simulink model "FP_250521"  (R2024a)
settings: Solver=VariableStepAuto  StartTime=0.0  StopTime=10.0  RelTol=1e-3
values from neighbouring files (symbols this model uses):
  global_path_xy_dense = [-80.8928520527 -80.3602143869 -79.8516651737 -79.3645247642 -78.8961135098 -78.4437517617 -78.004759871 -77.5764581893 -77.1561670675 -76.7412068571 -76.3288979094 -75.9165605754 ... (728 elements, 364x2)]    [global_path_xy_dense_y-34.mat]
undefined symbols (not defined in the file or in its folder): Do_waypoints, do_waypoints_tail_shifted, pathXY, route1_waypoint, route1_waypoint_raw, route2_waypoint, route2_waypoint_raw, route3_waypoint, route3_waypoint_raw
libraries: CarMaker4SL x192, slpidlib x4
(part 4 of 4)

== matlab function FP_250521/Final Project3/Scenario 1/MATLAB Function4  ==
  settings: updateMethod=DISCRETE  sampleTime=0.05
  data: waypoints input; local_waypoints_ output; vehicle_position input; head input
% function local_waypoints_ = global_to_local_waypoints(waypoints, vehicle_position, head)
%     N = size(waypoints, 1);
%     local_waypoints_ = zeros(N, 2);
% 
%     % 이동 평균 필터 윈도우 크기 설정
%     window_size = 65;
% 
% 
%     % 이동 평균 필터 적용 (x, y 각각)
%     x_filtered = movmean(waypoints(:,1), window_size);
%     y_filtered = movmean(waypoints(:,2), window_size);
% 
%     % 좌표계 변환을 위한 cos/sin
%     cos_yaw = cos(-head);
%     sin_yaw = sin(-head);
% 
%     for i = 1:N
%         dx = x_filtered(i) - vehicle_position(1);
%         dy = y_filtered(i) - vehicle_position(2);
% 
%         local_x = dx * cos_yaw - dy * sin_yaw;
%         local_y = dx * sin_yaw + dy * cos_yaw;
% 
%         local_waypoints_(i,1) = local_x;
%         local_waypoints_(i,2) = local_y;
%     end
% end

function local_waypoints_ = global_to_local_waypoints(waypoints, vehicle_position, head)
    N = size(waypoints, 1);
    local_waypoints_ = zeros(N, 2);

    window_size_main = 65;    % 기본 윈도우
    window_size_tail = 20;    % 꼬리(마지막 70개 구간) 윈도우

    x_filtered = zeros(N,1);
    y_filtered = zeros(N,1);

    for i = 1:N
        % 마지막 70개 전부터 윈도우 크기 30 적용
        if i > N - 70
            w = window_size_tail;
        else
            w = window_size_main;
        end
        % 윈도우 중앙 기준: [i - left, i + right] 범위
        half_win = floor(w/2);
        idx1 = max(1, i - half_win);
        idx2 = min(N, i + half_win);
        x_filtered(i) = mean(waypoints(idx1:idx2, 1));
        y_filtered(i) = mean(waypoints(idx1:idx2, 2));
    end

    % 좌표계 변환
    cos_yaw = cos(-head);
    sin_yaw = sin(-head);

    for i = 1:N
        dx = x_filtered(i) - vehicle_position(1);
        dy = y_filtered(i) - vehicle_position(2);

        local_x = dx * cos_yaw - dy * sin_yaw;
        local_y = dx * sin_yaw + dy * cos_yaw;

        local_waypoints_(i,1) = local_x;
        local_waypoints_(i,2) = local_y;
    end
end

== matlab function FP_250521/Final Project3/Scenario 1/MATLAB Function9 ==
  settings: updateMethod=DISCRETE  sampleTime=0.05
  data: ego_pos input; traffic_info input; ego_lane_idx output; wp1 input; wp2 input; wp3 input; traffic_lane_idx output
function [ego_lane_idx, traffic_lane_idx] = get_lane_indices_split(ego_pos, traffic_info, wp1, wp2, wp3)
% ego_pos: [1 x 2]
% traffic_info: [8 x 10] → 각 행: [x, y, vx, vy, ax, ay, yaw, yawRate, length, width]
% wp1~3: [N x 2] (차선별 waypoint 좌표)
% ego_lane_idx: 자차 차선 번호 (1~3)
% traffic_lane_idx: [8 x 1] (각 차량의 차선 번호)

    traffic_pos = traffic_info(:, 1:2);  % x, y 추출
    num_traffic = size(traffic_pos, 1);  % 8 expected
    traffic_lane_idx = zeros(num_traffic, 1);

    % 거리 계산 함수
    function d = min_dist(p, wp)
        dx = wp(:,1) - p(1);
        dy = wp(:,2) - p(2);
        d = min(sqrt(dx.^2 + dy.^2));
    end

    % 자차 차선 판단
    d1 = min_dist(ego_pos, wp1);
    d2 = min_dist(ego_pos, wp2);
    d3 = min_dist(ego_pos, wp3);
    [~, ego_lane_idx] = min([d1, d2, d3]);

    % 트래픽 차량들 차선 판단
    for i = 1:num_traffic
        car_pos = traffic_pos(i, :);
        d1 = min_dist(car_pos, wp1);
        d2 = min_dist(car_pos, wp2);
        d3 = min_dist(car_pos, wp3);
        [~, traffic_lane_idx(i)] = min([d1, d2, d3]);
    end
end

== matlab function FP_250521/Final Project3/Scenario 1/MATLAB Function ==
  data: u1 input; y output; u2 input
function y = and_logic_latch_permanent(u1, u2)
%#codegen
persistent latch;
if isempty(latch)
    latch = 0;
end

% 정지 조건에 한 번이라도 들어가면 latch=1이 되고, 이후엔 절대 복귀하지 않음
if (u1 > 5) && (u1 < 6) && (u2 > -38) && (u2 < -35)
    latch = 1;
end

y = latch;
end

== matlab function FP_250521/Final Project1/Scenario 1/MATLAB Function11 ==
  settings: updateMethod=DISCRETE  sampleTime=0.05
  data: ego_pos input; ego_yaw input; ego_vx input; ego_lane_idx input; traffic_info input; target_speed output; traffic_lane_idx input; debug_dist output
% function [target_speed, debug_dist] = acc_target_speed_global_based( ...
%     ego_pos, ego_yaw, ego_vx, ego_lane_idx, ...
%     traffic_info, traffic_lane_idx)
% 
%     % 기본 설정
%     default_speed = 16.0;   % m/s
%     min_gap = 20;           % 최소 안전 거리
%     max_gap = 35;           % 거리 완충 구간
% 
%     % === traffic_info: [8x10] ===
%     % 컬럼:
%     % 1: x, 2: y, 3: vx, 4: vy, 5: ax, 6: ay, 7: yaw, 8: yawrate, 9: len, 10: width
%     traffic_pos = traffic_info(:, 1:2);  % [8x2]
%     traffic_vx = traffic_info(:, 3);     % [8x1]
% 
%     L = size(traffic_info, 1);  % 차량 수 (8)
% 
%     min_dist = inf;
%     front_vx = 0;
%     found = false;
% 
%     % Ego 진행 방향 단위벡터
%     ego_dir = [cos(ego_yaw); sin(ego_yaw)];
% 
%     for i = 1:L
%         if traffic_lane_idx(i) == ego_lane_idx
%             dx = traffic_pos(i,1) - ego_pos(1);
%             dy = traffic_pos(i,2) - ego_pos(2);
%             rel_vec = [dx; dy];
% 
%             % 전방 차량인지 판단
%             if dot(rel_vec, ego_dir) > 0
%                 dist = norm(rel_vec);
% 
%                 if dist < min_dist
%                     min_dist = dist;
%                     front_vx = traffic_vx(i);
%                     found = true;
%                 end
%             end
%         end
%     end
% 
%     % 속도 설정
%     target_speed = default_speed;
% 
%     if found
%         if min_dist < min_gap
%             target_speed = front_vx;
%         elseif min_dist < max_gap
%             ratio = (min_dist - min_gap) / (max_gap - min_gap);
%             target_speed = front_vx * ratio + default_speed * (1 - ratio);
%         else
%             target_speed = default_speed;
%         end
%     end
% 
%     debug_dist = min_dist;
% end



function [target_speed, debug_dist] = acc_target_speed_global_based( ...
    ego_pos, ego_yaw, ego_vx, ego_lane_idx, ...
    traffic_info, traffic_lane_idx)

    % 기본 설정
    default_speed = 18;   % m/s
    min_gap = 25;           % 최소 안전 거리
    max_gap = 50;           % 거리 완충 구간
    min_speed = 3.5;        % 최저속도(정지 방지)

    % === traffic_info: [8x10] ===
    % 1: x, 2: y, 3: vx, ...
    traffic_pos = traffic_info(:, 1:2);  % [8x2]
    traffic_vx = traffic_info(:, 3);     % [8x1]

    L = size(traffic_info, 1);  % 차량 수 (8)

    min_dist = inf;
    front_vx = 0;
    found = false;

    % Ego 진행 방향 단위벡터
    ego_dir = [cos(ego_yaw); sin(ego_yaw)];

    for i = 1:L
        if traffic_lane_idx(i) == ego_lane_idx
            dx = traffic_pos(i,1) - ego_pos(1);
            dy = traffic_pos(i,2) - ego_pos(2);
            rel_vec = [dx; dy];

            % 전방 차량인지 판단
            if dot(rel_vec, ego_dir) > 0
                dist = norm(rel_vec);

                if dist < min_dist
                    min_dist = dist;
                    front_vx = traffic_vx(i);
                    found = true;
                end
            end
        end
    end

    % 속도 설정
    target_speed = default_speed;

    if found
        % *** 디버깅 로그 출력 (필요시 주석 해제) ***
        % disp(['front_vx=', num2str(front_vx), ', min_dist=', num2str(min_dist)]);

        % front_vx가 비정상(음수/NaN/이상치)이거나 너무 작으면 방어!
        if isnan(front_vx) || front_vx < 0
            front_vx = min_speed;
        end

        if min_dist < min_gap
            % 앞차 속도가 0일 때만 내 차도 정지, 그 외엔 최소 속도 유지
            if front_vx <= min_speed
                target_speed = min_speed;
            else
                target_speed = front_vx;
            end
        elseif min_dist < max_gap
            ratio = (min_dist - min_gap) / (max_gap - min_gap);
            % 보간 결과가 너무 작을 경우도 방어
            blend_speed = front_vx * ratio + default_speed * (1 - ratio);
            target_speed = max(blend_speed, min_speed);
        else
            target_speed = default_speed;
        end
    end

    % 추가 방어: target_speed는 항상 min_speed 이상 보장
    target_speed = max(target_speed, min_speed);

    debug_dist = min_dist;
end

== matlab function FP_250521/Final Project1/Scenario 1/MATLAB Function3 ==
  settings: updateMethod=DISCRETE  sampleTime=0.05
  data: poly_coeff input; lateral_error output; velocity input; lookahead_time input; x_lookahead output; delta_ff output; dy output; d2y output; kappa output
function [lateral_error, x_lookahead, delta_ff, dy, d2y, kappa] = compute_lateral_error_(poly_coeff, velocity, lookahead_time)
% ------------------------------------------------------------
% 경로 다항식 기반 곡률 및 조향각 계산 (스무딩 포함)
% Waypoint 부족 시 조향각 0 처리
% ------------------------------------------------------------

% 휠베이스
L = 3.0;

% Waypoint 부족으로 poly_coeff가 모두 0일 경우 → 계산 중단
if all(poly_coeff == 0)
    lateral_error = 0;
    x_lookahead = velocity * lookahead_time;
    delta_ff = 0;
    dy = 0;
    d2y = 0;
    kappa = 0;
    return;
end

% 다항식 계수 추출
a = 0; b = 0; c = 0; d = 0;
n = length(poly_coeff);
if n == 4
    a = poly_coeff(1); b = poly_coeff(2); c = poly_coeff(3); d = poly_coeff(4);
elseif n == 3
    b = poly_coeff(1); c = poly_coeff(2); d = poly_coeff(3);
elseif n == 2
    c = poly_coeff(1); d = poly_coeff(2);
else
    d = poly_coeff(1);
end

% 1. lateral error (x = 0)
lateral_error = d;

% 2. lookahead 위치
x_lookahead = velocity * lookahead_time;

% 3. dy, d2y
dy = 3*a*x_lookahead^2 + 2*b*x_lookahead + c;
d2y = 6*a*x_lookahead + 2*b;

% 4. kappa 계산 (수치 안정성 보장)
denominator = (1 + dy^2)^(3/2);
if denominator < 1e-6
    denominator = 1e-6;
end
kappa = d2y / denominator;

% 5. 조향각 계산
delta_now = L * kappa;

% 6. Moving Average Filter 적용 (스무딩)
persistent delta_buffer
if isempty(delta_buffer)
    delta_buffer = zeros(1, 30);  % 최근 30개 저장
end

% shift + 최신값 추가
delta_buffer = [delta_now, delta_buffer(1:end-1)];

% 평균값 출력
delta_ff = mean(delta_buffer);

end

== matlab function FP_250521/Final Project1/Scenario 1/MATLAB Function4 ==
  settings: updateMethod=DISCRETE  sampleTime=0.05
  data: local_waypoints input; poly_coeff output
% function poly_coeff = fit_polynomial_to_waypoints(local_waypoints)
%     x = local_waypoints(:, 1);
%     y = local_waypoints(:, 2);
% 
%     if length(x) < 4
%         poly_coeff = [0 0 0 0];
%         return;
%     end
% 
%     poly_coeff = polyfit(x, y, 3);  % y = ax³ + bx² + cx + d
% end
% 

function poly_coeff = fit_polynomial_to_waypoints_(local_waypoints)

% 설정값
poly_order = 3;
max_points = 10;
x_limit = 20;
y_limit = 5;

% 1. x > 0, x < x_limit, |y| < y_limit 필터링
idx = find( ...
    local_waypoints(:,1) > 0 & ...
    local_waypoints(:,1) < x_limit & ...
    abs(local_waypoints(:,2)) < y_limit );

filtered = local_waypoints(idx, :);

% 2. 앞쪽 max_points개만 사용
N = min(max_points, size(filtered, 1));
x = filtered(1:N, 1);
y = filtered(1:N, 2);

% 3. 피팅 수행
if length(x) >= poly_order + 1
    poly_coeff = polyfit(x, y, poly_order);
else
    poly_coeff = zeros(1, 4);
end

end

== matlab function FP_250521/Final Project1/Scenario 1/MATLAB Function4  ==
  settings: updateMethod=DISCRETE  sampleTime=0.05
  data: waypoints input; local_waypoints_ output; vehicle_position input; head input
function local_waypoints_ = global_to_local_waypoints(waypoints, vehicle_position, head)
    N = size(waypoints, 1);
    local_waypoints_ = zeros(N, 2);

    % 이동 평균 필터 윈도우 크기 설정
    window_size = 65;


    % 이동 평균 필터 적용 (x, y 각각)
    x_filtered = movmean(waypoints(:,1), window_size);
    y_filtered = movmean(waypoints(:,2), window_size);

    % 좌표계 변환을 위한 cos/sin
    cos_yaw = cos(-head);
    sin_yaw = sin(-head);

    for i = 1:N
        dx = x_filtered(i) - vehicle_position(1);
        dy = y_filtered(i) - vehicle_position(2);

        local_x = dx * cos_yaw - dy * sin_yaw;
        local_y = dx * sin_yaw + dy * cos_yaw;

        local_waypoints_(i,1) = local_x;
        local_waypoints_(i,2) = local_y;
    end
end

== matlab function FP_250521/Final Project1/Scenario 1/MATLAB Function9 ==
  settings: updateMethod=DISCRETE  sampleTime=0.05
  data: ego_pos input; traffic_info input; ego_lane_idx output; wp1 input; wp2 input; wp3 input; traffic_lane_idx output
function [ego_lane_idx, traffic_lane_idx] = get_lane_indices_split(ego_pos, traffic_info, wp1, wp2, wp3)
% ego_pos: [1 x 2]
% traffic_info: [8 x 10] → 각 행: [x, y, vx, vy, ax, ay, yaw, yawRate, length, width]
% wp1~3: [N x 2] (차선별 waypoint 좌표)
% ego_lane_idx: 자차 차선 번호 (1~3)
% traffic_lane_idx: [8 x 1] (각 차량의 차선 번호)

    traffic_pos = traffic_info(:, 1:2);  % x, y 추출
    num_traffic = size(traffic_pos, 1);  % 8 expected
    traffic_lane_idx = zeros(num_traffic, 1);

    % 거리 계산 함수
    function d = min_dist(p, wp)
        dx = wp(:,1) - p(1);
        dy = wp(:,2) - p(2);
        d = min(sqrt(dx.^2 + dy.^2));
    end

    % 자차 차선 판단
    d1 = min_dist(ego_pos, wp1);
    d2 = min_dist(ego_pos, wp2);
    d3 = min_dist(ego_pos, wp3);
    [~, ego_lane_idx] = min([d1, d2, d3]);

    % 트래픽 차량들 차선 판단
    for i = 1:num_traffic
        car_pos = traffic_pos(i, :);
        d1 = min_dist(car_pos, wp1);
        d2 = min_dist(car_pos, wp2);
        d3 = min_dist(car_pos, wp3);
        [~, traffic_lane_idx(i)] = min([d1, d2, d3]);
    end
end

== matlab function FP_250521/Final Project3/Scenario 1/MATLAB Function11 ==
  settings: updateMethod=DISCRETE  sampleTime=0.05
  data: ego_pos input; ego_yaw input; ego_vx input; ego_lane_idx input; traffic_info input; target_speed output; traffic_lane_idx input; debug_dist output; global_x input; stop_flag output
% function [target_speed, debug_dist] = acc_target_speed_global_based( ...
%     ego_pos, ego_yaw, ego_vx, ego_lane_idx, ...
%     traffic_info, traffic_lane_idx)
% 
%     % 기본 설정
%     default_speed = 16.0;   % m/s
%     min_gap = 20;           % 최소 안전 거리
%     max_gap = 35;           % 거리 완충 구간
% 
%     % === traffic_info: [8x10] ===
%     % 컬럼:
%     % 1: x, 2: y, 3: vx, 4: vy, 5: ax, 6: ay, 7: yaw, 8: yawrate, 9: len, 10: width
%     traffic_pos = traffic_info(:, 1:2);  % [8x2]
%     traffic_vx = traffic_info(:, 3);     % [8x1]
% 
%     L = size(traffic_info, 1);  % 차량 수 (8)
% 
%     min_dist = inf;
%     front_vx = 0;
%     found = false;
% 
%     % Ego 진행 방향 단위벡터
%     ego_dir = [cos(ego_yaw); sin(ego_yaw)];
% 
%     for i = 1:L
%         if traffic_lane_idx(i) == ego_lane_idx
%             dx = traffic_pos(i,1) - ego_pos(1);
%             dy = traffic_pos(i,2) - ego_pos(2);
%             rel_vec = [dx; dy];
% 
%             % 전방 차량인지 판단
%             if dot(rel_vec, ego_dir) > 0
%                 dist = norm(rel_vec);
% 
%                 if dist < min_dist
%                     min_dist = dist;
%                     front_vx = traffic_vx(i);
%                     found = true;
%                 end
%             end
%         end
%     end
% 
%     % 속도 설정
%     target_speed = default_speed;
% 
%     if found
%         if min_dist < min_gap
%             target_speed = front_vx;
%         elseif min_dist < max_gap
%             ratio = (min_dist - min_gap) / (max_gap - min_gap);
%             target_speed = front_vx * ratio + default_speed * (1 - ratio);
%         else
%             target_speed = default_speed;
%         end
%     end
% 
%     debug_dist = min_dist;
% end


% 
% function [target_speed, debug_dist] = acc_target_speed_global_based( ...
%     ego_pos, ego_yaw, ego_vx, ego_lane_idx, ...
%     traffic_info, traffic_lane_idx, stop_flag)
% 
%     % 기본 설정
%     default_speed = 3.0;   % m/s
%     min_gap = 25;           % 최소 안전 거리
%     max_gap = 50;           % 거리 완충 구간
%     min_speed = 3.0;        % 최저속도(정지 방지)
% 
%     % === traffic_info: [8x10] ===
%     % 1: x, 2: y, 3: vx, ...
%     traffic_pos = traffic_info(:, 1:2);  % [8x2]
%     traffic_vx = traffic_info(:, 3);     % [8x1]
% 
%     L = size(traffic_info, 1);  % 차량 수 (8)
% 
%     min_dist = inf;
%     front_vx = 0;
%     found = false;
% 
%     % Ego 진행 방향 단위벡터
%     ego_dir = [cos(ego_yaw); sin(ego_yaw)];
% 
%     for i = 1:L
%         if traffic_lane_idx(i) == ego_lane_idx
%             dx = traffic_pos(i,1) - ego_pos(1);
%             dy = traffic_pos(i,2) - ego_pos(2);
%             rel_vec = [dx; dy];
% 
%             % 전방 차량인지 판단
%             if dot(rel_vec, ego_dir) > 0
%                 dist = norm(rel_vec);
% 
%                 if dist < min_dist
%                     min_dist = dist;
%                     front_vx = traffic_vx(i);
%                     found = true;
%                 end
%             end
%         end
%     end
% 
%     % 속도 설정
%     target_speed = default_speed;
% 
%     if found
%         % *** 디버깅 로그 출력 (필요시 주석 해제) ***
%         % disp(['front_vx=', num2str(front_vx), ', min_dist=', num2str(min_dist)]);
% 
%         % front_vx가 비정상(음수/NaN/이상치)이거나 너무 작으면 방어!
%         if isnan(front_vx) || front_vx < 0
%             front_vx = min_speed;
%         end
% 
%         if min_dist < min_gap
%             % 앞차 속도가 0일 때만 내 차도 정지, 그 외엔 최소 속도 유지
%             if front_vx <= min_speed
%                 target_speed = min_speed;
%             else
%                 target_speed = front_vx;
%             end
%         elseif min_dist < max_gap
%             ratio = (min_dist - min_gap) / (max_gap - min_gap);
%             % 보간 결과가 너무 작을 경우도 방어
%             blend_speed = front_vx * ratio + default_speed * (1 - ratio);
%             target_speed = max(blend_speed, min_speed);
%         else
%             target_speed = default_speed;
%         end
%     end
% 
%     % 추가 방어: target_speed는 항상 min_speed 이상 보장
%     target_speed = max(target_speed, min_speed);
% 
%     % --- 정지 플래그가 1이면, 타겟 속도를 강제로 0 ---
%     if stop_flag == 1
%         target_speed = 0;
%     end
% 
%     debug_dist = min_dist;
% 
% 
% 
% 
% end




function [target_speed, debug_dist, stop_flag] = acc_target_speed_global_based( ...
    ego_pos, ego_yaw, ego_vx, ego_lane_idx, ...
    traffic_info, traffic_lane_idx, global_x)
% 래치형 stop_flag + 타겟 속도 제어
% global_x: 자차의 글로벌 X좌표 (정지 조건)
% ego_vx : 자차 속도 (m/s)

    % --- persistent stop_flag (래치 논리) ---
    persistent latched_stop;
    if isempty(latched_stop)
        latched_stop = 0;
    end

    % --- 정지 조건: 글로벌 x>8 이상이면 래치, 속도 0이면 해제 ---
    if (global_x > 8)
        latched_stop = 1;
    elseif (ego_vx < 0.01) % 실제로 완전히 멈춤(속도가 0이 되면) 해제
        latched_stop = 0;
    end
    stop_flag = latched_stop;

    % ===== 기존 타겟 속도 제어 로직 =====
    default_speed = 3.0;   % m/s
    min_gap = 25;
    max_gap = 50;
    min_speed = 3.0;

    traffic_pos = traffic_info(:, 1:2);
    traffic_vx = traffic_info(:, 3);

    L = size(traffic_info, 1);

    min_dist = inf;
    front_vx = 0;
    found = false;

    ego_dir = [cos(ego_yaw); sin(ego_yaw)];

    for i = 1:L
        if traffic_lane_idx(i) == ego_lane_idx
            dx = traffic_pos(i,1) - ego_pos(1);
            dy = traffic_pos(i,2) - ego_pos(2);
            rel_vec = [dx; dy];

            if dot(rel_vec, ego_dir) > 0
                dist = norm(rel_vec);

                if dist < min_dist
                    min_dist = dist;
                    front_vx = traffic_vx(i);
                    found = true;
                end
            end
        end
    end

    % 기본 속도 설정
    target_speed = default_speed;

    if found
        if isnan(front_vx) || front_vx < 0
            front_vx = min_speed;
        end

        if min_dist < min_gap
            if front_vx <= min_speed
                target_speed = min_speed;
            else
                target_speed = front_vx;
            end
        elseif min_dist < max_gap
            ratio = (min_dist - min_gap) / (max_gap - min_gap);
            blend_speed = front_vx * ratio + default_speed * (1 - ratio);
            target_speed = max(blend_speed, min_speed);
        else
            target_speed = default_speed;
        end
    end

    % 추가 방어: target_speed는 항상 min_speed 이상 보장
    target_speed = max(target_speed, min_speed);

    % --- 정지 래치 적용: stop_flag가 1이면, 무조건 0 ---
    if stop_flag == 1
        target_speed = 0;
    end

    debug_dist = min_dist;
end
